simulink model "PX01s"  (R2015b)
settings: Solver=VariableStepAuto  StartTime=0.0  StopTime=10.0  RelTol=1e-3
libraries: fl_lib x19, nesl_utility x3
settings Model: Creator=xmax1946  LastModifiedBy=xmax1946

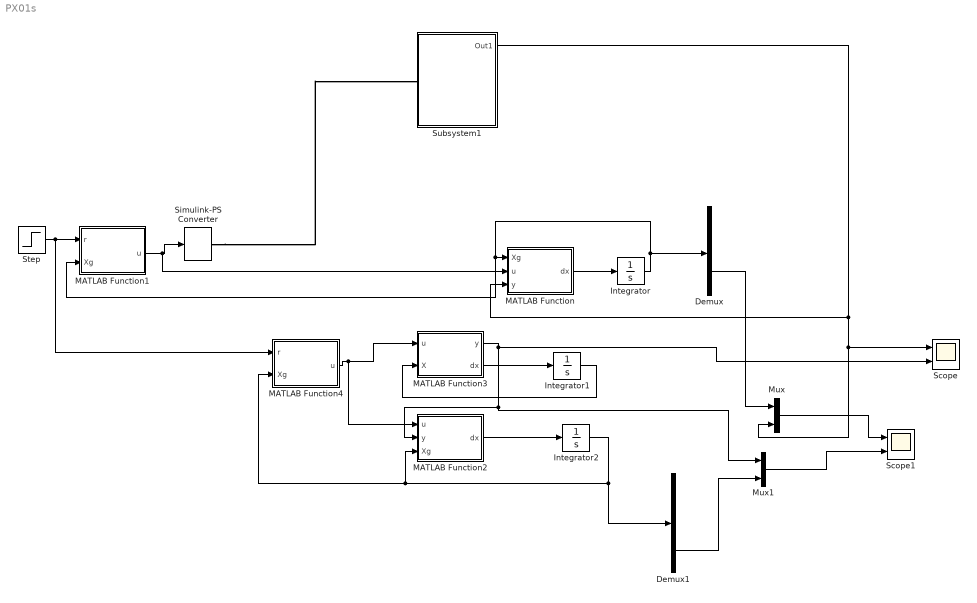
== system PX01s ==
  Demux : Demux  Outputs=6
  Demux1 : Demux  Outputs=6
  Integrator : Integrator  InitialCondition=[1;1;1;1;1;1]
  Integrator1 : Integrator  InitialCondition=[0;0;0;0;0;0]  IgnoreLimit=on
  Integrator2 : Integrator  InitialCondition=[1;1;1;1;1;1]
  MATLAB Function : MATLAB Function  TreatAsAtomicUnit=on
  MATLAB Function1 : MATLAB Function  TreatAsAtomicUnit=on
  MATLAB Function2 : MATLAB Function  TreatAsAtomicUnit=on
  MATLAB Function3 : MATLAB Function  TreatAsAtomicUnit=on
  MATLAB Function4 : MATLAB Function  TreatAsAtomicUnit=on
  Mux : Mux  Inputs=2
  Mux1 : Mux  Inputs=2
  Scope : Scope  NumInputPorts=2
  Scope1 : Scope  NumInputPorts=2
  Simulink-PS Converter : nesl_utility/Simulink-PS Converter  PhysicalDomain=network_engine_domain  SubClassName=ps_input  LeftPortType=input  RightPortType=output  PseudoPeriodic=off  Frequencies=[]  NoiseDistribution=none  NoiseParameters=[]  Unit=1  AffineConversion=off  InputFiltering=off  SimscapeFilterOrder=1  InputFilterTimeConstant=0.001  UdotUserProvided=1
  Step : Step  SampleTime=0
  Subsystem1 : Subsystem
  wires:
  MATLAB Function/1(dx) -> Integrator/1
  Integrator/1 -> MATLAB Function1/2(Xg), MATLAB Function/1(Xg), Demux/1
  Step/1 -> MATLAB Function4/1(r), MATLAB Function1/1(r)
  MATLAB Function1/1(u) -> MATLAB Function/2(u), Simulink-PS Converter/1
  MATLAB Function4/1(u) -> MATLAB Function2/1(u), MATLAB Function3/1(u)
  MATLAB Function2/1(dx) -> Integrator2/1
  MATLAB Function3/2(dx) -> Integrator1/1
  Integrator1/1 -> MATLAB Function3/2(X)
  Integrator2/1 -> Demux1/1, MATLAB Function4/2(Xg), MATLAB Function2/3(Xg)
  MATLAB Function3/1(y) -> Scope/2, Mux1/1, MATLAB Function2/2(y)
  Mux/1 -> Scope1/1
  Mux1/1 -> Scope1/2
  Subsystem1/1(Out1) -> Mux/2, Scope/1, MATLAB Function/3(y)
  Demux/5 -> Mux/1
  Demux1/5 -> Mux1/2
  connections:
  Simulink-PS Converter/RConn1 -- Subsystem1/LConn1

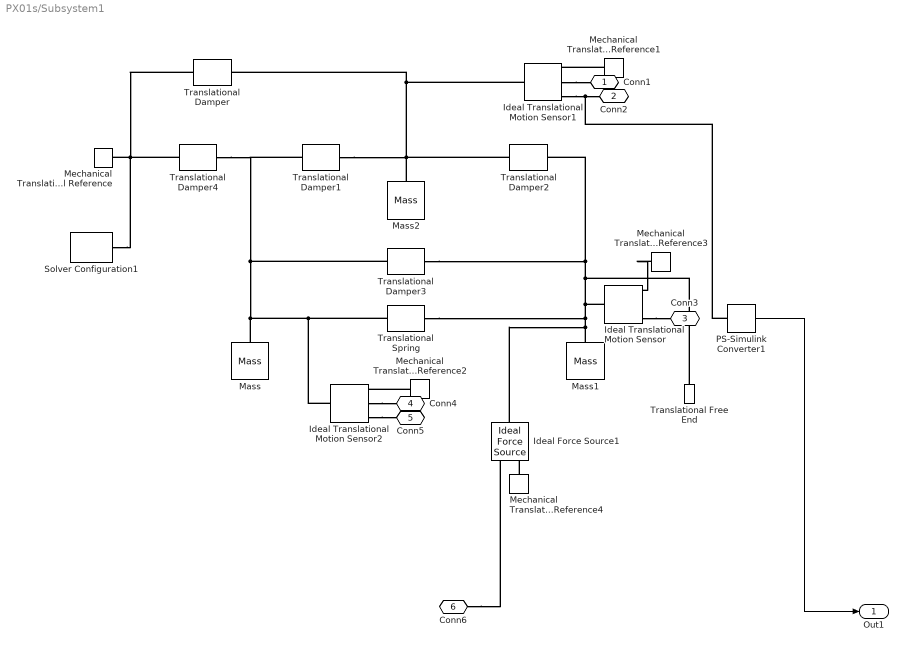
== system PX01s/Subsystem1 ==
  Ideal Force Source1 : fl_lib/Mechanical/Mechanical Sources/Ideal Force Source
  Ideal Translational Motion Sensor : fl_lib/Mechanical/Mechanical Sensors/Ideal Translational Motion Sensor  offset=0 m
  Ideal Translational Motion Sensor1 : fl_lib/Mechanical/Mechanical Sensors/Ideal Translational Motion Sensor  offset=0 m
  Ideal Translational Motion Sensor2 : fl_lib/Mechanical/Mechanical Sensors/Ideal Translational Motion Sensor  offset=0 m
  Mass : fl_lib/Mechanical/Translational Elements/Mass  mass=2 kg  v_specify=off  v_priority=None  v=0 m/s  f_specify=off  f_priority=None  f=0 N
  Mass1 : fl_lib/Mechanical/Translational Elements/Mass  mass=1 kg  v_specify=off  v_priority=None  v=0 m/s  f_specify=off  f_priority=None  f=0 N
  Mass2 : fl_lib/Mechanical/Translational Elements/Mass  mass=1 kg  v_specify=off  v_priority=None  v=0 m/s  f_specify=off  f_priority=None  f=0 N
  Mechanical Translational Reference{,1..4} (5 alike) : fl_lib/Mechanical/Translational Elements/Mechanical Translational Reference
  PS-Simulink Converter1 : nesl_utility/PS-Simulink Converter  PhysicalDomain=network_engine_domain  SubClassName=ps_output  LeftPortType=input  RightPortType=output  PseudoPeriodic=off  Frequencies=[]  Unit=1  AffineConversion=off
  Solver Configuration1 : nesl_utility/Solver Configuration  PhysicalDomain=network_engine_domain  SubClassName=solver  LeftPortType=input  RightPortType=generic  Accelerate=off  Tones=[]  Harmonics=[]  SimulateNoise=off  Profile=off  UseLocalSampling=off  EnableSwitchedLinearOptims=on  FrequencyDomain=off  UseCCode=off  RelTol=0.001  AbsTol=1e-06  MinStep=1e-09  ToWorkspace=off  RevertToSquareIcSolve=off  NumHomotopyIterations=100  PhasorMode=off  PhasorModeNumHarmonics=1  DoDC=off  ResidualTolerance=1e-09  UseLocalSolver=off  LocalSolverChoice=NE_BACKWARD_EULER_ADVANCER  LocalSolverSampleTime=0.001  DoFixedCost=off  MaxNonlinIter=3  MaxModeIter=2  LinearAlgebra=Sparse  DelaysMemoryBudget=1024  AutomaticFiltering=on  FilteringTimeConstant=0.001
  Translational Damper{,1..4} (5 alike) : fl_lib/Mechanical/Translational Elements/Translational Damper  D=1 N/(m/s)  v_specify=off  v_priority=None  v=0 m/s  f_specify=off  f_priority=None  f=0 N
  Translational Free End : fl_lib/Mechanical/Translational Elements/Translational Free End  v_specify=off  v_priority=None  v=0 m/s
  Translational Spring : fl_lib/Mechanical/Translational Elements/Translational Spring  spr_rate=2 N/m  v_specify=off  v_priority=None  v=0 m/s  f_specify=off  f_priority=None  f=0 N  x_specify=off  x_priority=None  x=0 m
  Conn1 : PMIOPort  Port=1  Side=Right
  Conn2 : PMIOPort  Port=2  Side=Right
  Conn3 : PMIOPort  Port=3  Side=Right
  Conn4 : PMIOPort  Port=4  Side=Right
  Conn5 : PMIOPort  Port=5  Side=Right
  Conn6 : PMIOPort  Port=6  Side=Left
  Out1 : Outport
  wires:
  PS-Simulink Converter1/1 -> Out1/1
  connections:
  Mechanical Translational Reference3/LConn1 -- Ideal Translational Motion Sensor/RConn1
  Conn6/RConn1 -- Ideal Force Source1/RConn1
  Mechanical Translational Reference1/LConn1 -- Ideal Translational Motion Sensor1/RConn1
  Mechanical Translational Reference2/LConn1 -- Ideal Translational Motion Sensor2/RConn1
  Mechanical Translational Reference4/LConn1 -- Ideal Force Source1/RConn2
  Mass1/LConn1 -- Ideal Force Source1/LConn1 -- Translational Spring/RConn1 -- Ideal Translational Motion Sensor/LConn1 -- Translational Damper3/RConn1 -- Translational Damper2/RConn1 -- Translational Free End/LConn1
  Mass2/LConn1 -- Translational Damper2/LConn1 -- Translational Damper1/RConn1 -- Ideal Translational Motion Sensor1/LConn1 -- Translational Damper/RConn1
  Ideal Translational Motion Sensor2/LConn1 -- Mass/LConn1 -- Translational Damper4/RConn1 -- Translational Damper1/LConn1 -- Translational Damper3/LConn1 -- Translational Spring/LConn1
  Translational Damper4/LConn1 -- Translational Damper/LConn1 -- Mechanical Translational Reference/LConn1 -- Solver Configuration1/RConn1
  Ideal Translational Motion Sensor2/RConn2 -- Conn4/RConn1
  Ideal Translational Motion Sensor1/RConn2 -- Conn1/RConn1
  Ideal Translational Motion Sensor2/RConn3 -- Conn5/RConn1
  Ideal Translational Motion Sensor1/RConn3 -- PS-Simulink Converter1/LConn1 -- Conn2/RConn1
  Ideal Translational Motion Sensor/RConn3 -- Conn3/RConn1

== matlab function PX01s/MATLAB Function1 ==
  data: r input; u output; Xg input
function u = fcn(r,Xg)
K=[5.2500    6.5000    3.2500    3.5000    3.2500    3.2500];
u=r-K*Xg;

== matlab function PX01s/MATLAB Function ==
  data: dx output; Xg input; u input; y input
function dx  = fss(Xg,u,y)
m1=2;
m2=1;
m3=1;
v1=1;
v2=1;
v3=1;
v4=1;
v5=1;
k=2;

A=[0,1,0,0,0,0;
  -k/m1,(-v2-v4-v1)/m1,k/m1,v2/m1,0,v4/m1
  0,0,0,1,0,0 
  k/m2,v2/m2,-k/m2,(-v2-v5)/m2,0,v5/m2
  0,0,0,0,0,1
  0,v4/m3,0,v5/m3,0,(-v4-v3-v5)/m3
    ];
 B=[0;0;0;1/m2;0;0];
 C=[0,0,0,0,1,0];
 L=[47.25;496.625;-521.5;65.75;18.5;115.25];
 dx=A*Xg+B*u+L*(y-C*Xg);

== matlab function PX01s/MATLAB Function2 ==
  data: u input; y input; Xg input; dx output
function dx  = fcn(u,y,Xg)
m1=2;
m2=1;
m3=1;
v1=1;
v2=1;
v3=1;
v4=1;
v5=1;
k=2;

A=[0,1,0,0,0,0;
  -k/m1,(-v2-v4-v1)/m1,k/m1,v2/m1,0,v4/m1
  0,0,0,1,0,0 
  k/m2,v2/m2,-k/m2,(-v2-v5)/m2,0,v5/m2
  0,0,0,0,0,1
  0,v4/m3,0,v5/m3,0,(-v4-v3-v5)/m3
    ];
B=[0;0;0;1/m2;0;0];
C=[0,0,0,0,1,0];
L=[47.25;496.625;-521.5;65.75;18.5;115.25];
dx=A*Xg+B*u+L*(y-C*Xg);

== matlab function PX01s/MATLAB Function3 ==
  data: u input; y output; X input; dx output
function [y,dx] = fcn(u,X)
m1=2;
m2=1;
m3=1;
v1=1;
v2=1;
v3=1;
v4=1;
v5=1;
k=2;

A=[0,1,0,0,0,0;
  -k/m1,(-v2-v4-v1)/m1,k/m1,v2/m1,0,v4/m1
  0,0,0,1,0,0 
  k/m2,v2/m2,-k/m2,(-v2-v5)/m2,0,v5/m2
  0,0,0,0,0,1
  0,v4/m3,0,v5/m3,0,(-v4-v3-v5)/m3
    ];
B=[0;0;0;1/m2;0;0];
C=[0,0,0,0,1,0];

dx=A*X+B*u;
y=C*X;

== matlab function PX01s/MATLAB Function4 ==
  data: r input; u output; Xg input
function u = fcn(r,Xg)
K=[5.2500    6.5000    3.2500    3.5000    3.2500    3.2500];
u=r-K*Xg;
